simulink model "Book6141"  (R2019b)
settings: Solver=ode4  StartTime=0.001  StopTime=10.0  FixedStep=0.001  RelTol=1e-3
settings Model: Creator=user  LastModifiedBy=user

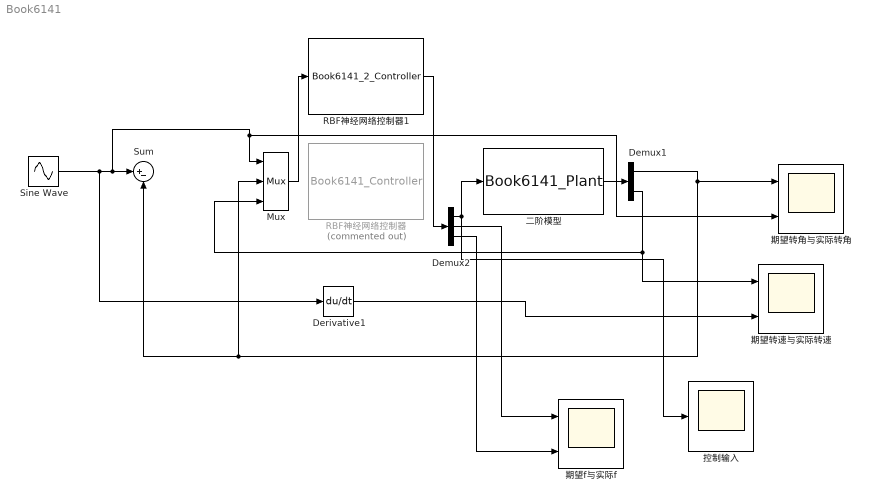
== system Book6141 ==
  Demux1 : Demux  Outputs=2
  Demux2 : Demux  Outputs=3
  Derivative1 : Derivative
  Mux : Mux  Inputs=3
  RBF神经网络控制器 : S-Function  Commented=on  FunctionName=Book6141_Controller  SFunctionDeploymentMode=off  EnableBusSupport=off
  RBF神经网络控制器1 : S-Function  FunctionName=Book6141_2_Controller  SFunctionDeploymentMode=off  EnableBusSupport=off
  Sine Wave : Sin  SampleTime=0
  Sum : Sum  Inputs=|+-
  二阶模型 : S-Function  FunctionName=Book6141_Plant  SFunctionDeploymentMode=off  EnableBusSupport=off
  控制输入 : Scope
  期望f与实际f : Scope  NumInputPorts=2
  期望转角与实际转角 : Scope  NumInputPorts=2
  期望转速与实际转速 : Scope  NumInputPorts=2
  wires:
  Sine Wave/1 -> Derivative1/1, Mux/1, 期望转角与实际转角/2, Sum/1
  Mux/1 -> RBF神经网络控制器1/1
  RBF神经网络控制器1/1 -> Demux2/1
  Derivative1/1 -> 期望转速与实际转速/2
  二阶模型/1 -> Demux1/1
  Demux1/2 -> Mux/3, 期望转速与实际转速/1
  Demux2/3 -> 期望f与实际f/2
  Demux2/1 -> 控制输入/1, 二阶模型/1
  Demux2/2 -> 期望f与实际f/1
  Demux1/1 -> Mux/2, Sum/2, 期望转角与实际转角/1
